simulink model "F16"  (R2024b)
settings: Solver=VariableStepAuto  StartTime=0.0  StopTime=10.0  RelTol=1e-3
values from neighbouring files (symbols this model uses):
  U = [10; 2; 0; 5; 2; 20]    [main.m]
  Y0 = [100; 4; 1; 0.1; 0.05; 0.08; 5; 0; 10; 0; 0; -200]    [main.m]
undefined symbols (not defined in the file or in its folder): F16_deq
settings Model: Creator=deepa  LastModifiedBy=deepa

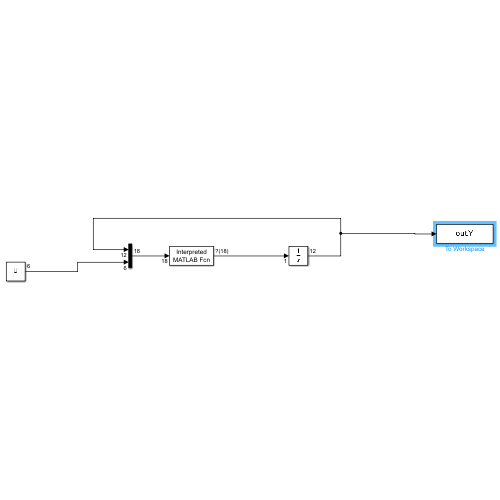
[thumbnail: Simulink's stored preview of the top-level diagram]
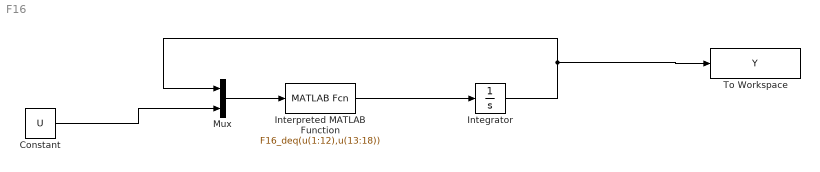
== system F16 ==
  Constant : Constant  Value=U
  Integrator : Integrator  InitialCondition=Y0
  Interpreted MATLAB Function : MATLABFcn  MATLABFcn=F16_deq(u(1:12),u(13:18))  Output1D=off
  Mux : Mux  Inputs=2
  To Workspace : ToWorkspace  VariableName=Y  SaveFormat=Timeseries  SampleTime=-1
  wires:
  Interpreted MATLAB Function/1 -> Integrator/1
  Integrator/1 -> Mux/1, To Workspace/1
  Constant/1 -> Mux/2
  Mux/1 -> Interpreted MATLAB Function/1
